simulink model "sra2_2"  (R2016a)
settings: Solver=ode45  StartTime=0.0  StopTime=30  RelTol=1e-5
values from neighbouring files (symbols this model uses):
  a1 = 0    [program2.m]    (also in program3.m = Hpcd.den{1}(2))
  a2 = 6.23    [program2.m]
  b = -291.8    [program2.m]    (also in program3.m = Hpcd.num{1}(3)/Hpcd.num{1}(2))
  c1 = c    (= 6)    [program2.m]
  c2 = (c1+1)/a2+0.1    (= 1.22359550562)    [program2.m]
  delta = 0.1    [program2.m]
  ftilda = 1000    [program2.m]
  Ti = 0.1605    [program2.m]
libraries: simulink x1
settings Model: Creator=andrei  LastModifiedBy=andrei

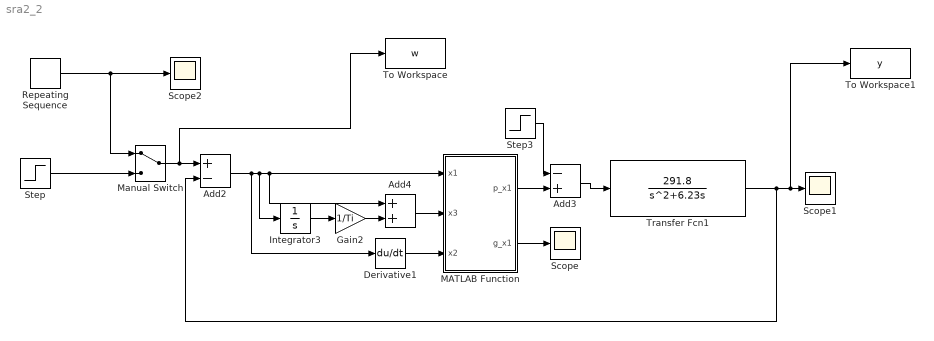
== system sra2_2 ==
  Add2 : Sum  Inputs=+-
  Add3 : Sum  Inputs=-+
  Add4 : Sum
  Derivative1 : Derivative
  Gain2 : Gain  Gain=1/Ti
  Integrator3 : Integrator
  MATLAB Function : MATLAB Function  TreatAsAtomicUnit=on
  Manual Switch : ManualSwitch
  Repeating Sequence : simulink/Sources/Repeating Sequence  rep_seq_t=[0.0001 5 5.0001 10 10.0001]  rep_seq_y=[0.0001 0.0000 5 5 5]
  Scope : Scope
  Scope1 : Scope
  Scope2 : Scope
  Step : Step  Time=0  SampleTime=0
  Step3 : Step  Time=7.5  After=0.01  SampleTime=0
  To Workspace : ToWorkspace  VariableName=w  SaveFormat=Timeseries  SampleTime=-1
  To Workspace1 : ToWorkspace  VariableName=y  SaveFormat=Timeseries  SampleTime=-1
  Transfer Fcn1 : TransferFcn  Numerator=[291.8]  Denominator=[1 6.23 0]
  wires:
  MATLAB Function/2(g_x1) -> Scope/1
  Add2/1 -> Integrator3/1, Add4/1, MATLAB Function/1(x1), Derivative1/1
  Repeating Sequence/1 -> Manual Switch/1, Scope2/1
  Step/1 -> Manual Switch/2
  Manual Switch/1 -> To Workspace/1, Add2/1
  Transfer Fcn1/1 -> Add2/2, To Workspace1/1, Scope1/1
  Derivative1/1 -> MATLAB Function/3(x2)
  Add4/1 -> MATLAB Function/2(x3)
  Gain2/1 -> Add4/2
  Integrator3/1 -> Gain2/1
  MATLAB Function/1(p_x1) -> Add3/2
  Add3/1 -> Transfer Fcn1/1
  Step3/1 -> Add3/1

== matlab function sra2_2/MATLAB Function ==
  data: x1 input; x3 input; p_x1 output; x2 input; c1 parameter; a1 parameter; a2 parameter; ftilda parameter; delta parameter; b parameter; Ti parameter; c2 parameter; g_x1 output
function [p_x1,g_x1] = fcn(x1,x3,x2,c1,a1, a2, ftilda, delta, b, Ti, c2)

alfa=(abs(((c1*c1-c1*c2*a2+c2*c2*a1+c1)/c2-1/Ti)*x1/c2+(c1-c2*a2+1)/(c2*c2)*x3)+ftilda)/(abs(b*x1))+delta;

g_x1=(c1*x1+c2*x2+x3)*x1;

p_x1=alfa*sign(g_x1)*x1;

end
